simulink model "ANN_model"  (R2023a)
settings: Solver=VariableStepAuto  StartTime=0.0  StopTime=T_e  RelTol=1e-3
libraries: neural x61, spspowerguiLib x1
(part 2 of 2)

== system ANN_model/Custom Neural Network/Layer 4/Delays 1 ==
  "p{4}" : Inport  PortDimensions=10
      mask Display: e = 0.06;c1 = [120 230 180]/255;c2 = ([120 230 180]+0)/(256+128);c3 = ([120 230 180]+128)/(256+128);patch([0 1 1 0],[0 0 1 1],c1);patch([0 1 1 1-e 1-e 0+e],[0 0 1 1-e 0+e 0+e],c2);patch([0 0 1 1-e 0+e 0+e],[0 1 1 1-e 1-e 0+e],c3);plot([0 1 1 0 0],[0 0 1 1 0]);
  mux : Mux  Inputs=1
      mask Display: e = 0.06;c1 = [120 150 230]/255;c2 = ([120 150 230]+0)/383;c3 = ([120 150 230]+128)/383;patch([0 1 1 0],[0 0 1 1],c1);patch([0 1 1 1-e 1-e 0+e],[0 0 1 1-e 0+e 0+e],c2);patch([0 0 1 1-e 0+e 0+e],[0 1 1 1-e 1-e 0+e],c3);plot([0 1 1 0 0],[0 0 1 1 0]);disp('Mux')
  "pd{4,3}" : Outport
      mask Display: e = 0.06;c1 = [120 230 180]/255;c2 = ([120 230 180]+0)/(256+128);c3 = ([120 230 180]+128)/(256+128);patch([0 1 1 0],[0 0 1 1],c1);patch([0 1 1 1-e 1-e 0+e],[0 0 1 1-e 0+e 0+e],c2);patch([0 0 1 1-e 0+e 0+e],[0 1 1 1-e 1-e 0+e],c3);plot([0 1 1 0 0],[0 0 1 1 0]);
  wires:
  "p{4}"/1 -> mux/1
  mux/1 -> "pd{4,3}"/1

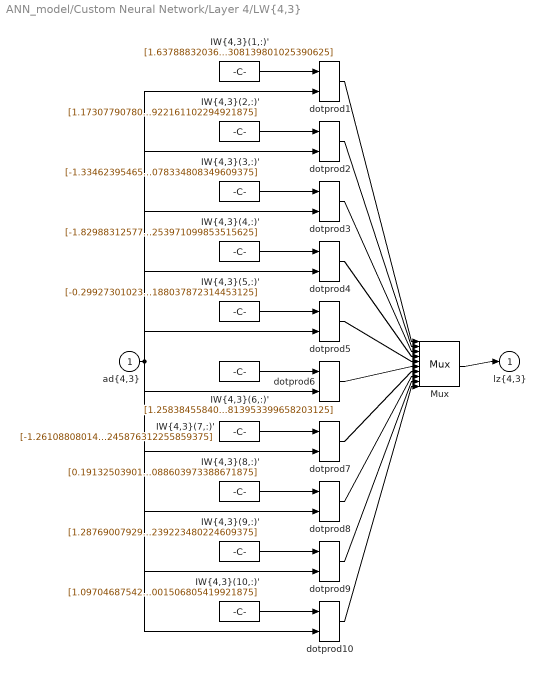
== system ANN_model/Custom Neural Network/Layer 4/LW{4,3} ==
  "ad{4,3}" : Inport  PortDimensions=10
      mask Display: e = 0.06;c1 = [120 230 180]/255;c2 = ([120 230 180]+0)/(256+128);c3 = ([120 230 180]+128)/(256+128);patch([0 1 1 0],[0 0 1 1],c1);patch([0 1 1 1-e 1-e 0+e],[0 0 1 1-e 0+e 0+e],c2);patch([0 0 1 1-e 0+e 0+e],[0 1 1 1-e 1-e 0+e],c3);plot([0 1 1 0 0],[0 0 1 1 0]);
  "IW{4,3}(1,:)'" : Constant  Value=[1.6378883203698550996563199078082107007503509521484375;0.7785713160290177459188498687581159174442291259765625;-3.134049077427762508563091614632867276668548583984375;-4.11400321800767354574190903804264962673187255859375;2.7023166374114051535570979467593133449554443359375;2.178799747279068554917103028856217861175537109375;-1.4904773301039540012169481997261755168437957763671875;-0.434657325226812718543811797644593752920627593994140625;-2.093640295600631251460299608879722654819488525390625;-0.4795777947227544135699872640543617308139801025390625]
      mask Display: e = 0.06;c1 = [120 150 230]/255;c2 = ([120 150 230]+0)/383;c3 = ([120 150 230]+128)/383;patch([0 1 1 0],[0 0 1 1],c1);patch([0 1 1 1-e 1-e 0+e],[0 0 1 1-e 0+e 0+e],c2);patch([0 0 1 1-e 0+e 0+e],[0 1 1 1-e 1-e 0+e],c3);plot([0 1 1 0 0],[0 0 1 1 0]);disp('weights');
  "IW{4,3}(10,:)'" : Constant  Value=[1.0970468754208211326073296731919981539249420166015625;2.598662475604209820545520415180362761020660400390625;3.47585894555124585991734420531429350376129150390625;0.23212021853686748418255092474282719194889068603515625;1.839725276361742434261259404593147337436676025390625;-0.05368765037105353854496314625066588632762432098388671875;2.278073107192821300515106486272998154163360595703125;-0.0687948159269435033369433085681521333754062652587890625;2.86853608695433859310242041829042136669158935546875;-0.328379018423550383953823939009453170001506805419921875]
      mask Display: e = 0.06;c1 = [120 150 230]/255;c2 = ([120 150 230]+0)/383;c3 = ([120 150 230]+128)/383;patch([0 1 1 0],[0 0 1 1],c1);patch([0 1 1 1-e 1-e 0+e],[0 0 1 1-e 0+e 0+e],c2);patch([0 0 1 1-e 0+e 0+e],[0 1 1 1-e 1-e 0+e],c3);plot([0 1 1 0 0],[0 0 1 1 0]);disp('weights');
  "IW{4,3}(2,:)'" : Constant  Value=[1.1730779078006194904304493320523761212825775146484375;-0.93733423397561865808569336877553723752498626708984375;1.4591051184685588371081621517078019678592681884765625;2.1481638705161412161714906687848269939422607421875;-0.97618086283236815692276877598487772047519683837890625;-1.2190160274977539511809254690888337790966033935546875;-1.2100782358443884501042475676513276994228363037109375;-2.800884352505108143560619282652623951435089111328125;0.394266235416011967540583782465546391904354095458984375;0.334912766900543779069465699649299494922161102294921875]
      mask Display: e = 0.06;c1 = [120 150 230]/255;c2 = ([120 150 230]+0)/383;c3 = ([120 150 230]+128)/383;patch([0 1 1 0],[0 0 1 1],c1);patch([0 1 1 1-e 1-e 0+e],[0 0 1 1-e 0+e 0+e],c2);patch([0 0 1 1-e 0+e 0+e],[0 1 1 1-e 1-e 0+e],c3);plot([0 1 1 0 0],[0 0 1 1 0]);disp('weights');
  "IW{4,3}(3,:)'" : Constant  Value=[-1.33462395465049876719376698019914329051971435546875;1.8839799879032177454263319305027835071086883544921875;3.681472741353296829203145534847863018512725830078125;1.707180142477845219417531552608124911785125732421875;-1.44817415107770131044162553735077381134033203125;-3.233967749450946893574609930510632693767547607421875;-1.7261889438801041318782836242462508380413055419921875;-1.873091929612898720591829260229133069515228271484375;0.85833257953746822099816426998586393892765045166015625;1.9157726496007574379376592332846485078334808349609375]
      mask Display: e = 0.06;c1 = [120 150 230]/255;c2 = ([120 150 230]+0)/383;c3 = ([120 150 230]+128)/383;patch([0 1 1 0],[0 0 1 1],c1);patch([0 1 1 1-e 1-e 0+e],[0 0 1 1-e 0+e 0+e],c2);patch([0 0 1 1-e 0+e 0+e],[0 1 1 1-e 1-e 0+e],c3);plot([0 1 1 0 0],[0 0 1 1 0]);disp('weights');
  "IW{4,3}(4,:)'" : Constant  Value=[-1.8298831257738987776662042961106635630130767822265625;-3.1645191260748770645250260713510215282440185546875;-1.2881244508082720923169972593314014375209808349609375;-0.493910555575517218329650859232060611248016357421875;-0.82949048138147596365143954244558699429035186767578125;0.69421918940789650864786608508438803255558013916015625;-1.844328494029690457267633973970077931880950927734375;1.5905908738831155968540542744449339807033538818359375;-1.66302593735684478559733179281465709209442138671875;1.22518832395793797473970698774792253971099853515625]
      mask Display: e = 0.06;c1 = [120 150 230]/255;c2 = ([120 150 230]+0)/383;c3 = ([120 150 230]+128)/383;patch([0 1 1 0],[0 0 1 1],c1);patch([0 1 1 1-e 1-e 0+e],[0 0 1 1-e 0+e 0+e],c2);patch([0 0 1 1-e 0+e 0+e],[0 1 1 1-e 1-e 0+e],c3);plot([0 1 1 0 0],[0 0 1 1 0]);disp('weights');
  "IW{4,3}(5,:)'" : Constant  Value=[-0.299273010230704128442624778472236357629299163818359375;0.50978913541735881853611545011517591774463653564453125;1.097906791329425590930668477085418999195098876953125;2.74186807520239117508253912092186510562896728515625;-0.71921684098344318414319786825217306613922119140625;-2.130424327935024120250773194129578769207000732421875;-0.48862893519710814960177458488033153116703033447265625;1.1831422162157119171155272852047346532344818115234375;0.119131740649917772234545054743648506700992584228515625;0.876286678272823582602768510696478188037872314453125]
      mask Display: e = 0.06;c1 = [120 150 230]/255;c2 = ([120 150 230]+0)/383;c3 = ([120 150 230]+128)/383;patch([0 1 1 0],[0 0 1 1],c1);patch([0 1 1 1-e 1-e 0+e],[0 0 1 1-e 0+e 0+e],c2);patch([0 0 1 1-e 0+e 0+e],[0 1 1 1-e 1-e 0+e],c3);plot([0 1 1 0 0],[0 0 1 1 0]);disp('weights');
  "IW{4,3}(6,:)'" : Constant  Value=[1.258384558409598952266605920158326625823974609375;-2.15265133408728370767448723199777305126190185546875;0.349871100632710818612025605034432373940944671630859375;0.17845212127078780017797043910832144320011138916015625;4.278098869715069696439968538470566272735595703125;-1.2651860443286204738200240171863697469234466552734375;-0.0431755036074752684971400640279171057045459747314453125;0.069751845298305970022312294531730003654956817626953125;-0.320437074873093863391915192551095969974994659423828125;-1.0338974588446216973380842318874783813953399658203125]
      mask Display: e = 0.06;c1 = [120 150 230]/255;c2 = ([120 150 230]+0)/383;c3 = ([120 150 230]+128)/383;patch([0 1 1 0],[0 0 1 1],c1);patch([0 1 1 1-e 1-e 0+e],[0 0 1 1-e 0+e 0+e],c2);patch([0 0 1 1-e 0+e 0+e],[0 1 1 1-e 1-e 0+e],c3);plot([0 1 1 0 0],[0 0 1 1 0]);disp('weights');
  "IW{4,3}(7,:)'" : Constant  Value=[-1.26108808014402828945321743958629667758941650390625;1.2982991534359396013087462051771581172943115234375;-0.35594753368714038277431654933025129139423370361328125;-0.13297185436369274302847998114884831011295318603515625;0.85757738162091190492475334394839592278003692626953125;0.87046854879330248788704693652107380330562591552734375;-3.2413727160328438259284666855819523334503173828125;-0.72558623336712846363383278003311716020107269287109375;0.10456892822654194341591704642269178293645381927490234375;-0.71452112693072178384312564958236180245876312255859375]
      mask Display: e = 0.06;c1 = [120 150 230]/255;c2 = ([120 150 230]+0)/383;c3 = ([120 150 230]+128)/383;patch([0 1 1 0],[0 0 1 1],c1);patch([0 1 1 1-e 1-e 0+e],[0 0 1 1-e 0+e 0+e],c2);patch([0 0 1 1-e 0+e 0+e],[0 1 1 1-e 1-e 0+e],c3);plot([0 1 1 0 0],[0 0 1 1 0]);disp('weights');
  "IW{4,3}(8,:)'" : Constant  Value=[0.1913250390145461443669461232275352813303470611572265625;0.225036006872918414867257297373726032674312591552734375;-6.11190586376111699706825675093568861484527587890625;1.1475267565847711015436516390764154493808746337890625;0.353383174212771600242177783002262003719806671142578125;6.0150369989034704332198089105077087879180908203125;1.605029225551447336073351834784261882305145263671875;0.49390716034623871610875767146353609859943389892578125;1.7498661214561515020449178337003104388713836669921875;2.643356415682688531632038575480692088603973388671875]
      mask Display: e = 0.06;c1 = [120 150 230]/255;c2 = ([120 150 230]+0)/383;c3 = ([120 150 230]+128)/383;patch([0 1 1 0],[0 0 1 1],c1);patch([0 1 1 1-e 1-e 0+e],[0 0 1 1-e 0+e 0+e],c2);patch([0 0 1 1-e 0+e 0+e],[0 1 1 1-e 1-e 0+e],c3);plot([0 1 1 0 0],[0 0 1 1 0]);disp('weights');
  "IW{4,3}(9,:)'" : Constant  Value=[1.287690079297733714014384531765244901180267333984375;-1.444902682493584666900687807356007397174835205078125;-0.29402508747429190183453329154872335493564605712890625;0.0264921265303505355792612618870407459326088428497314453125;-0.12147051106321561653178520145957008935511112213134765625;-0.382550265942154743559200369418249465525150299072265625;-0.7916339264109328865970383048988878726959228515625;-1.8418305905607745831531474323128350079059600830078125;-0.56450801436953546019736904781893827021121978759765625;-0.98129506363542906566266310619539581239223480224609375]
      mask Display: e = 0.06;c1 = [120 150 230]/255;c2 = ([120 150 230]+0)/383;c3 = ([120 150 230]+128)/383;patch([0 1 1 0],[0 0 1 1],c1);patch([0 1 1 1-e 1-e 0+e],[0 0 1 1-e 0+e 0+e],c2);patch([0 0 1 1-e 0+e 0+e],[0 1 1 1-e 1-e 0+e],c3);plot([0 1 1 0 0],[0 0 1 1 0]);disp('weights');
  Mux : Mux  Inputs=10
      mask Display: e = 0.06;c1 = [120 150 230]/255;c2 = ([120 150 230]+0)/383;c3 = ([120 150 230]+128)/383;patch([0 1 1 0],[0 0 1 1],c1);patch([0 1 1 1-e 1-e 0+e],[0 0 1 1-e 0+e 0+e],c2);patch([0 0 1 1-e 0+e 0+e],[0 1 1 1-e 1-e 0+e],c3);plot([0 1 1 0 0],[0 0 1 1 0]);disp('Mux');
  dotprod{1..10} (10 alike) : neural/Weight Functions/dotprod
  "lz{4,3}" : Outport
      mask Display: e = 0.06;c1 = [120 230 180]/255;c2 = ([120 230 180]+0)/(256+128);c3 = ([120 230 180]+128)/(256+128);patch([0 1 1 0],[0 0 1 1],c1);patch([0 1 1 1-e 1-e 0+e],[0 0 1 1-e 0+e 0+e],c2);patch([0 0 1 1-e 0+e 0+e],[0 1 1 1-e 1-e 0+e],c3);plot([0 1 1 0 0],[0 0 1 1 0]);
  wires:
  "IW{4,3}(1,:)'"/1 -> dotprod1/1
  "ad{4,3}"/1 -> dotprod1/2, dotprod2/2, dotprod3/2, dotprod4/2, dotprod5/2, dotprod6/2, dotprod7/2, dotprod8/2, dotprod9/2, dotprod10/2
  dotprod1/1 -> Mux/1
  "IW{4,3}(2,:)'"/1 -> dotprod2/1
  dotprod2/1 -> Mux/2
  "IW{4,3}(3,:)'"/1 -> dotprod3/1
  dotprod3/1 -> Mux/3
  "IW{4,3}(4,:)'"/1 -> dotprod4/1
  dotprod4/1 -> Mux/4
  "IW{4,3}(5,:)'"/1 -> dotprod5/1
  dotprod5/1 -> Mux/5
  "IW{4,3}(6,:)'"/1 -> dotprod6/1
  dotprod6/1 -> Mux/6
  "IW{4,3}(7,:)'"/1 -> dotprod7/1
  dotprod7/1 -> Mux/7
  "IW{4,3}(8,:)'"/1 -> dotprod8/1
  dotprod8/1 -> Mux/8
  "IW{4,3}(9,:)'"/1 -> dotprod9/1
  dotprod9/1 -> Mux/9
  "IW{4,3}(10,:)'"/1 -> dotprod10/1
  dotprod10/1 -> Mux/10
  Mux/1 -> "lz{4,3}"/1

== system ANN_model/Custom Neural Network/Layer 5/Delays 1 ==
  "p{5}" : Inport  PortDimensions=10
      mask Display: e = 0.06;c1 = [120 230 180]/255;c2 = ([120 230 180]+0)/(256+128);c3 = ([120 230 180]+128)/(256+128);patch([0 1 1 0],[0 0 1 1],c1);patch([0 1 1 1-e 1-e 0+e],[0 0 1 1-e 0+e 0+e],c2);patch([0 0 1 1-e 0+e 0+e],[0 1 1 1-e 1-e 0+e],c3);plot([0 1 1 0 0],[0 0 1 1 0]);
  mux : Mux  Inputs=1
      mask Display: e = 0.06;c1 = [120 150 230]/255;c2 = ([120 150 230]+0)/383;c3 = ([120 150 230]+128)/383;patch([0 1 1 0],[0 0 1 1],c1);patch([0 1 1 1-e 1-e 0+e],[0 0 1 1-e 0+e 0+e],c2);patch([0 0 1 1-e 0+e 0+e],[0 1 1 1-e 1-e 0+e],c3);plot([0 1 1 0 0],[0 0 1 1 0]);disp('Mux')
  "pd{5,4}" : Outport
      mask Display: e = 0.06;c1 = [120 230 180]/255;c2 = ([120 230 180]+0)/(256+128);c3 = ([120 230 180]+128)/(256+128);patch([0 1 1 0],[0 0 1 1],c1);patch([0 1 1 1-e 1-e 0+e],[0 0 1 1-e 0+e 0+e],c2);patch([0 0 1 1-e 0+e 0+e],[0 1 1 1-e 1-e 0+e],c3);plot([0 1 1 0 0],[0 0 1 1 0]);
  wires:
  "p{5}"/1 -> mux/1
  mux/1 -> "pd{5,4}"/1

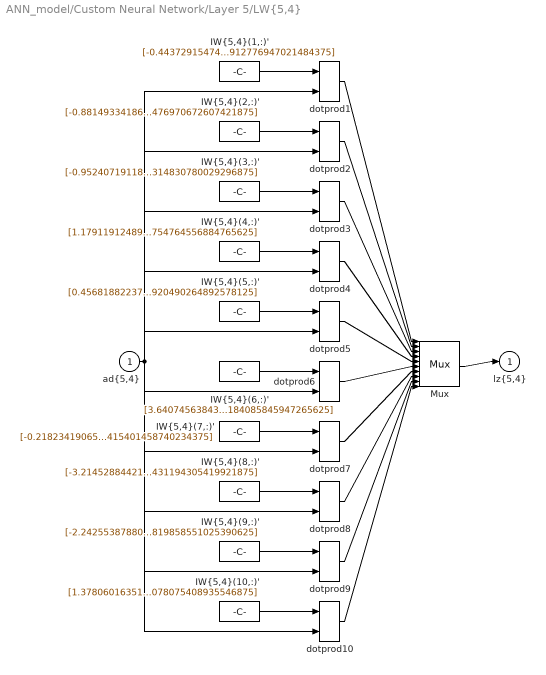
== system ANN_model/Custom Neural Network/Layer 5/LW{5,4} ==
  "ad{5,4}" : Inport  PortDimensions=10
      mask Display: e = 0.06;c1 = [120 230 180]/255;c2 = ([120 230 180]+0)/(256+128);c3 = ([120 230 180]+128)/(256+128);patch([0 1 1 0],[0 0 1 1],c1);patch([0 1 1 1-e 1-e 0+e],[0 0 1 1-e 0+e 0+e],c2);patch([0 0 1 1-e 0+e 0+e],[0 1 1 1-e 1-e 0+e],c3);plot([0 1 1 0 0],[0 0 1 1 0]);
  "IW{5,4}(1,:)'" : Constant  Value=[-0.44372915474945251457228323488379828631877899169921875;-0.08048856572732365766142947904882021248340606689453125;0.3052289457363439595383169944398105144500732421875;-1.592886200917619898831389946280978620052337646484375;-1.0574976706712602148030555326840840280055999755859375;3.0318441877980557563887487049214541912078857421875;2.6572457807686422626147759729065001010894775390625;0.285644863788504010937430166450212709605693817138671875;2.545513406488022045692787287407554686069488525390625;2.398794400241926805250614052056334912776947021484375]
      mask Display: e = 0.06;c1 = [120 150 230]/255;c2 = ([120 150 230]+0)/383;c3 = ([120 150 230]+128)/383;patch([0 1 1 0],[0 0 1 1],c1);patch([0 1 1 1-e 1-e 0+e],[0 0 1 1-e 0+e 0+e],c2);patch([0 0 1 1-e 0+e 0+e],[0 1 1 1-e 1-e 0+e],c3);plot([0 1 1 0 0],[0 0 1 1 0]);disp('weights');
  "IW{5,4}(10,:)'" : Constant  Value=[1.378060163511015456805353096569888293743133544921875;-3.192256397588707717005718222935684025287628173828125;0.7384007420041598379611968994140625;-0.53648879404282912020107687567360699176788330078125;1.9022303694091338144289693445898592472076416015625;-0.409782401405845042585696091919089667499065399169921875;-3.154158555223784521359675636631436645984649658203125;-0.8081742825994415735380016485578380525112152099609375;-1.55348612712726374951444086036644876003265380859375;-2.46842866002258443103301033261232078075408935546875]
      mask Display: e = 0.06;c1 = [120 150 230]/255;c2 = ([120 150 230]+0)/383;c3 = ([120 150 230]+128)/383;patch([0 1 1 0],[0 0 1 1],c1);patch([0 1 1 1-e 1-e 0+e],[0 0 1 1-e 0+e 0+e],c2);patch([0 0 1 1-e 0+e 0+e],[0 1 1 1-e 1-e 0+e],c3);plot([0 1 1 0 0],[0 0 1 1 0]);disp('weights');
  "IW{5,4}(2,:)'" : Constant  Value=[-0.88149334186260841494942042118054814636707305908203125;-0.85890941940042087043849505789694376289844512939453125;-0.401436754943303275577903832527226768434047698974609375;-1.134388757481453513520364140276797115802764892578125;1.6701735466533638163610930860158987343311309814453125;5.81019966239588736556243020459078252315521240234375;3.2797891234911400459850483457557857036590576171875;-0.84227492066083053945391156958066858351230621337890625;-4.382743717276245121183819719590246677398681640625;-1.533996205454193795247874732012860476970672607421875]
      mask Display: e = 0.06;c1 = [120 150 230]/255;c2 = ([120 150 230]+0)/383;c3 = ([120 150 230]+128)/383;patch([0 1 1 0],[0 0 1 1],c1);patch([0 1 1 1-e 1-e 0+e],[0 0 1 1-e 0+e 0+e],c2);patch([0 0 1 1-e 0+e 0+e],[0 1 1 1-e 1-e 0+e],c3);plot([0 1 1 0 0],[0 0 1 1 0]);disp('weights');
  "IW{5,4}(3,:)'" : Constant  Value=[-0.9524071911833764669808033431763760745525360107421875;-1.440247864426563939588277207803912460803985595703125;-0.09067337052139878839085440631606616079807281494140625;3.211647447886596840049833190278150141239166259765625;-3.113299611645719000563303779927082359790802001953125;0.277171941789911946418811794501380063593387603759765625;-0.914863066338964525670007787994109094142913818359375;-0.374506231519017962483530936879105865955352783203125;-2.186056986813969427174697557347826659679412841796875;1.6900012467605936006265210380661301314830780029296875]
      mask Display: e = 0.06;c1 = [120 150 230]/255;c2 = ([120 150 230]+0)/383;c3 = ([120 150 230]+128)/383;patch([0 1 1 0],[0 0 1 1],c1);patch([0 1 1 1-e 1-e 0+e],[0 0 1 1-e 0+e 0+e],c2);patch([0 0 1 1-e 0+e 0+e],[0 1 1 1-e 1-e 0+e],c3);plot([0 1 1 0 0],[0 0 1 1 0]);disp('weights');
  "IW{5,4}(4,:)'" : Constant  Value=[1.1791191248966408355869361912482418119907379150390625;2.031207704811440084569085229304619133472442626953125;0.1341964448633394535459473217997583560645580291748046875;-0.99291564480543481607810463174246251583099365234375;1.2426211118028354096765042413608171045780181884765625;-0.048657784134124505703855589899831102229654788970947265625;-1.18748455604717850775386978057213127613067626953125;-0.659011772753751667863753027631901204586029052734375;-2.255847322448911729253495650482363998889923095703125;-1.068045974981336687648081351653672754764556884765625]
      mask Display: e = 0.06;c1 = [120 150 230]/255;c2 = ([120 150 230]+0)/383;c3 = ([120 150 230]+128)/383;patch([0 1 1 0],[0 0 1 1],c1);patch([0 1 1 1-e 1-e 0+e],[0 0 1 1-e 0+e 0+e],c2);patch([0 0 1 1-e 0+e 0+e],[0 1 1 1-e 1-e 0+e],c3);plot([0 1 1 0 0],[0 0 1 1 0]);disp('weights');
  "IW{5,4}(5,:)'" : Constant  Value=[0.45681882237817117431433189267409034073352813720703125;0.2191730373466506953672450208614463917911052703857421875;-0.1898345875871349786034869566719862632453441619873046875;-1.0656921974338160463702251945505850017070770263671875;1.027043662399730106216111380490474402904510498046875;-2.1421702478158888283132910146377980709075927734375;-1.3597015711374342838979600855964235961437225341796875;-0.32682144504051524602772360594826750457286834716796875;1.7764736465346384619579112040810286998748779296875;-1.7639521181190709331332300280337221920490264892578125]
      mask Display: e = 0.06;c1 = [120 150 230]/255;c2 = ([120 150 230]+0)/383;c3 = ([120 150 230]+128)/383;patch([0 1 1 0],[0 0 1 1],c1);patch([0 1 1 1-e 1-e 0+e],[0 0 1 1-e 0+e 0+e],c2);patch([0 0 1 1-e 0+e 0+e],[0 1 1 1-e 1-e 0+e],c3);plot([0 1 1 0 0],[0 0 1 1 0]);disp('weights');
  "IW{5,4}(6,:)'" : Constant  Value=[3.640745638430612274305531173013150691986083984375;-1.4278802970870696498195684398524463176727294921875;2.9485922999351661388800494023598730564117431640625;-4.41275925093963561351984026259742677211761474609375;4.30707915728340839933707684394903481006622314453125;7.9507897478846825123355301911942660808563232421875;5.16378772799802998605400716769509017467498779296875;-1.0149200969258249660498449884471483528614044189453125;-1.0426889523547802074432411245652474462985992431640625;-0.7695055887698549756947841160581447184085845947265625]
      mask Display: e = 0.06;c1 = [120 150 230]/255;c2 = ([120 150 230]+0)/383;c3 = ([120 150 230]+128)/383;patch([0 1 1 0],[0 0 1 1],c1);patch([0 1 1 1-e 1-e 0+e],[0 0 1 1-e 0+e 0+e],c2);patch([0 0 1 1-e 0+e 0+e],[0 1 1 1-e 1-e 0+e],c3);plot([0 1 1 0 0],[0 0 1 1 0]);disp('weights');
  "IW{5,4}(7,:)'" : Constant  Value=[-0.2182341906556131139183207778842188417911529541015625;0.08219980701825425895012955379570485092699527740478515625;-0.5711068151788041280525476395268924534320831298828125;-0.66723523270064044599081398700946010649204254150390625;0.545520924027612874596115943859331309795379638671875;-0.7218856964225783823252413640148006379604339599609375;-0.354626208286069000141793594593764282763004302978515625;-0.147860903080202887860394866947899572551250457763671875;-1.053609900673512900226569399819709360599517822265625;-0.42586212762334818560105986762209795415401458740234375]
      mask Display: e = 0.06;c1 = [120 150 230]/255;c2 = ([120 150 230]+0)/383;c3 = ([120 150 230]+128)/383;patch([0 1 1 0],[0 0 1 1],c1);patch([0 1 1 1-e 1-e 0+e],[0 0 1 1-e 0+e 0+e],c2);patch([0 0 1 1-e 0+e 0+e],[0 1 1 1-e 1-e 0+e],c3);plot([0 1 1 0 0],[0 0 1 1 0]);disp('weights');
  "IW{5,4}(8,:)'" : Constant  Value=[-3.214528844219887826483272874611429870128631591796875;-2.95747394430882426519247019314207136631011962890625;-2.636002696425631341980988509021699428558349609375;2.571593011677298701300742322928272187709808349609375;2.46358558223354151550665847025811672210693359375;-1.4523946986657636504247648190357722342014312744140625;4.22796835534398951494949869811534881591796875;-1.024206817104519107175519820884801447391510009765625;7.0624384896016412227481851004995405673980712890625;-6.86198307148493835683211727882735431194305419921875]
      mask Display: e = 0.06;c1 = [120 150 230]/255;c2 = ([120 150 230]+0)/383;c3 = ([120 150 230]+128)/383;patch([0 1 1 0],[0 0 1 1],c1);patch([0 1 1 1-e 1-e 0+e],[0 0 1 1-e 0+e 0+e],c2);patch([0 0 1 1-e 0+e 0+e],[0 1 1 1-e 1-e 0+e],c3);plot([0 1 1 0 0],[0 0 1 1 0]);disp('weights');
  "IW{5,4}(9,:)'" : Constant  Value=[-2.24255387880731671401690618949942290782928466796875;0.2131474041792032758646513457279070280492305755615234375;-0.11451107992129962165339662760743522085249423980712890625;-0.058408580933412897195911028802584041841328144073486328125;-6.67116050890009137930292126839049160480499267578125;1.186492100019120865539434817037545144557952880859375;0.66577299553018309818952502610045485198497772216796875;0.0212200176263356195260900705079620820470154285430908203125;1.1533073803396529655174163053743541240692138671875;-0.3195905918601855688621071749366819858551025390625]
      mask Display: e = 0.06;c1 = [120 150 230]/255;c2 = ([120 150 230]+0)/383;c3 = ([120 150 230]+128)/383;patch([0 1 1 0],[0 0 1 1],c1);patch([0 1 1 1-e 1-e 0+e],[0 0 1 1-e 0+e 0+e],c2);patch([0 0 1 1-e 0+e 0+e],[0 1 1 1-e 1-e 0+e],c3);plot([0 1 1 0 0],[0 0 1 1 0]);disp('weights');
  Mux : Mux  Inputs=10
      mask Display: e = 0.06;c1 = [120 150 230]/255;c2 = ([120 150 230]+0)/383;c3 = ([120 150 230]+128)/383;patch([0 1 1 0],[0 0 1 1],c1);patch([0 1 1 1-e 1-e 0+e],[0 0 1 1-e 0+e 0+e],c2);patch([0 0 1 1-e 0+e 0+e],[0 1 1 1-e 1-e 0+e],c3);plot([0 1 1 0 0],[0 0 1 1 0]);disp('Mux');
  dotprod{1..10} (10 alike) : neural/Weight Functions/dotprod
  "lz{5,4}" : Outport
      mask Display: e = 0.06;c1 = [120 230 180]/255;c2 = ([120 230 180]+0)/(256+128);c3 = ([120 230 180]+128)/(256+128);patch([0 1 1 0],[0 0 1 1],c1);patch([0 1 1 1-e 1-e 0+e],[0 0 1 1-e 0+e 0+e],c2);patch([0 0 1 1-e 0+e 0+e],[0 1 1 1-e 1-e 0+e],c3);plot([0 1 1 0 0],[0 0 1 1 0]);
  wires:
  "IW{5,4}(1,:)'"/1 -> dotprod1/1
  "ad{5,4}"/1 -> dotprod1/2, dotprod2/2, dotprod3/2, dotprod4/2, dotprod5/2, dotprod6/2, dotprod7/2, dotprod8/2, dotprod9/2, dotprod10/2
  dotprod1/1 -> Mux/1
  "IW{5,4}(2,:)'"/1 -> dotprod2/1
  dotprod2/1 -> Mux/2
  "IW{5,4}(3,:)'"/1 -> dotprod3/1
  dotprod3/1 -> Mux/3
  "IW{5,4}(4,:)'"/1 -> dotprod4/1
  dotprod4/1 -> Mux/4
  "IW{5,4}(5,:)'"/1 -> dotprod5/1
  dotprod5/1 -> Mux/5
  "IW{5,4}(6,:)'"/1 -> dotprod6/1
  dotprod6/1 -> Mux/6
  "IW{5,4}(7,:)'"/1 -> dotprod7/1
  dotprod7/1 -> Mux/7
  "IW{5,4}(8,:)'"/1 -> dotprod8/1
  dotprod8/1 -> Mux/8
  "IW{5,4}(9,:)'"/1 -> dotprod9/1
  dotprod9/1 -> Mux/9
  "IW{5,4}(10,:)'"/1 -> dotprod10/1
  dotprod10/1 -> Mux/10
  Mux/1 -> "lz{5,4}"/1

== system ANN_model/Custom Neural Network/Layer 6/Delays 1 ==
  "p{6}" : Inport  PortDimensions=10
      mask Display: e = 0.06;c1 = [120 230 180]/255;c2 = ([120 230 180]+0)/(256+128);c3 = ([120 230 180]+128)/(256+128);patch([0 1 1 0],[0 0 1 1],c1);patch([0 1 1 1-e 1-e 0+e],[0 0 1 1-e 0+e 0+e],c2);patch([0 0 1 1-e 0+e 0+e],[0 1 1 1-e 1-e 0+e],c3);plot([0 1 1 0 0],[0 0 1 1 0]);
  mux : Mux  Inputs=1
      mask Display: e = 0.06;c1 = [120 150 230]/255;c2 = ([120 150 230]+0)/383;c3 = ([120 150 230]+128)/383;patch([0 1 1 0],[0 0 1 1],c1);patch([0 1 1 1-e 1-e 0+e],[0 0 1 1-e 0+e 0+e],c2);patch([0 0 1 1-e 0+e 0+e],[0 1 1 1-e 1-e 0+e],c3);plot([0 1 1 0 0],[0 0 1 1 0]);disp('Mux')
  "pd{6,5}" : Outport
      mask Display: e = 0.06;c1 = [120 230 180]/255;c2 = ([120 230 180]+0)/(256+128);c3 = ([120 230 180]+128)/(256+128);patch([0 1 1 0],[0 0 1 1],c1);patch([0 1 1 1-e 1-e 0+e],[0 0 1 1-e 0+e 0+e],c2);patch([0 0 1 1-e 0+e 0+e],[0 1 1 1-e 1-e 0+e],c3);plot([0 1 1 0 0],[0 0 1 1 0]);
  wires:
  "p{6}"/1 -> mux/1
  mux/1 -> "pd{6,5}"/1

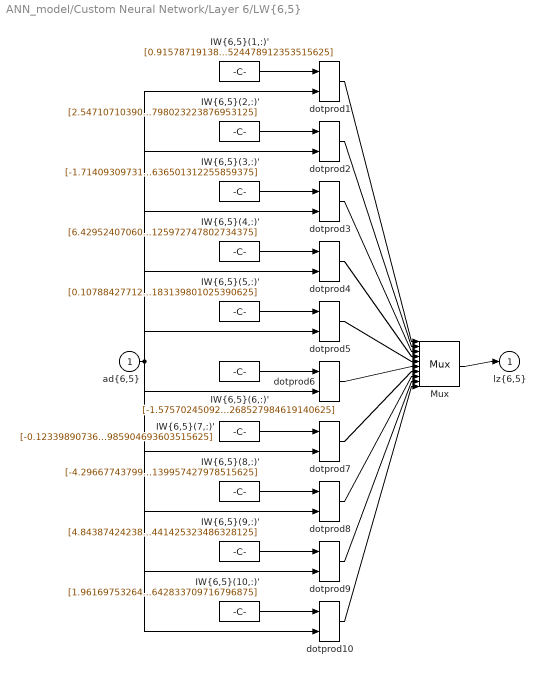
== system ANN_model/Custom Neural Network/Layer 6/LW{6,5} ==
  "ad{6,5}" : Inport  PortDimensions=10
      mask Display: e = 0.06;c1 = [120 230 180]/255;c2 = ([120 230 180]+0)/(256+128);c3 = ([120 230 180]+128)/(256+128);patch([0 1 1 0],[0 0 1 1],c1);patch([0 1 1 1-e 1-e 0+e],[0 0 1 1-e 0+e 0+e],c2);patch([0 0 1 1-e 0+e 0+e],[0 1 1 1-e 1-e 0+e],c3);plot([0 1 1 0 0],[0 0 1 1 0]);
  "IW{6,5}(1,:)'" : Constant  Value=[0.91578719138092001816886522647109813988208770751953125;-1.55629738752322754891110889730043709278106689453125;0.54686041367531867951612412070971913635730743408203125;2.748536495852894834257540424005128443241119384765625;-0.69203669557024827252433851754176430404186248779296875;0.1562862665844011733629059790473547764122486114501953125;-1.1030783465285132205480067568714730441570281982421875;-0.0231553801418886047447376341779090580530464649200439453125;2.756258727328901425579488204675726592540740966796875;-0.48193857734411393867191009121597744524478912353515625]
      mask Display: e = 0.06;c1 = [120 150 230]/255;c2 = ([120 150 230]+0)/383;c3 = ([120 150 230]+128)/383;patch([0 1 1 0],[0 0 1 1],c1);patch([0 1 1 1-e 1-e 0+e],[0 0 1 1-e 0+e 0+e],c2);patch([0 0 1 1-e 0+e 0+e],[0 1 1 1-e 1-e 0+e],c3);plot([0 1 1 0 0],[0 0 1 1 0]);disp('weights');
  "IW{6,5}(10,:)'" : Constant  Value=[1.9616975326464112239222004063776694238185882568359375;-1.0899447413761318426139723669621162116527557373046875;1.2031767189375008886287332643405534327030181884765625;2.03906650011060630589554421021603047847747802734375;2.50600129434051144272643796284683048725128173828125;0.4252173926274915860545888790511526167392730712890625;-2.230662929131254745840351461083628237247467041015625;-0.07630327116655109820353430905015557073056697845458984375;-1.3079000135828906525858883469481952488422393798828125;-1.4236777433878973209147034140187315642833709716796875]
      mask Display: e = 0.06;c1 = [120 150 230]/255;c2 = ([120 150 230]+0)/383;c3 = ([120 150 230]+128)/383;patch([0 1 1 0],[0 0 1 1],c1);patch([0 1 1 1-e 1-e 0+e],[0 0 1 1-e 0+e 0+e],c2);patch([0 0 1 1-e 0+e 0+e],[0 1 1 1-e 1-e 0+e],c3);plot([0 1 1 0 0],[0 0 1 1 0]);disp('weights');
  "IW{6,5}(2,:)'" : Constant  Value=[2.547107103900183577849247740232385694980621337890625;-1.2370150361727978438608488431782461702823638916015625;0.989661630898456490257331097382120788097381591796875;-2.862189591738488303462872863747179508209228515625;-1.8002999427067949422820447580306790769100189208984375;-1.071065879591814873350585912703536450862884521484375;-0.357942338977107532560495428697322495281696319580078125;-0.474367748873758376948472914591548033058643341064453125;-2.868888218359867181561639881692826747894287109375;0.59131397526320317314940666619804687798023223876953125]
      mask Display: e = 0.06;c1 = [120 150 230]/255;c2 = ([120 150 230]+0)/383;c3 = ([120 150 230]+128)/383;patch([0 1 1 0],[0 0 1 1],c1);patch([0 1 1 1-e 1-e 0+e],[0 0 1 1-e 0+e 0+e],c2);patch([0 0 1 1-e 0+e 0+e],[0 1 1 1-e 1-e 0+e],c3);plot([0 1 1 0 0],[0 0 1 1 0]);disp('weights');
  "IW{6,5}(3,:)'" : Constant  Value=[-1.7140930973196975006800357732572592794895172119140625;0.1535266433030496868727965420475811697542667388916015625;-1.584619785562153548852393214474432170391082763671875;0.72668287956691279827481366737629286944866180419921875;0.032179627298217404474112157686249702237546443939208984375;-0.225522758623212860040752048007561825215816497802734375;0.1636206551172376955083365146492724306881427764892578125;-0.00968246359250476452962264062307440326549112796783447265625;0.34861364819909079759696624023490585386753082275390625;0.56444552208853548957989687551162205636501312255859375]
      mask Display: e = 0.06;c1 = [120 150 230]/255;c2 = ([120 150 230]+0)/383;c3 = ([120 150 230]+128)/383;patch([0 1 1 0],[0 0 1 1],c1);patch([0 1 1 1-e 1-e 0+e],[0 0 1 1-e 0+e 0+e],c2);patch([0 0 1 1-e 0+e 0+e],[0 1 1 1-e 1-e 0+e],c3);plot([0 1 1 0 0],[0 0 1 1 0]);disp('weights');
  "IW{6,5}(4,:)'" : Constant  Value=[6.429524070607516961217697826214134693145751953125;-2.74197592228397990510302406619302928447723388671875;0.256586162676969486984290824693744070827960968017578125;0.97924535689561176265982567201717756688594818115234375;-0.048702914274068032085551749332807958126068115234375;1.1089893356618187869599978512269444763660430908203125;0.18199381171876527485409269502270035445690155029296875;-1.6772060408506941353579122733208350837230682373046875;-1.4422098408455801266114804093376733362674713134765625;-0.70564252785975634107984433285309933125972747802734375]
      mask Display: e = 0.06;c1 = [120 150 230]/255;c2 = ([120 150 230]+0)/383;c3 = ([120 150 230]+128)/383;patch([0 1 1 0],[0 0 1 1],c1);patch([0 1 1 1-e 1-e 0+e],[0 0 1 1-e 0+e 0+e],c2);patch([0 0 1 1-e 0+e 0+e],[0 1 1 1-e 1-e 0+e],c3);plot([0 1 1 0 0],[0 0 1 1 0]);disp('weights');
  "IW{6,5}(5,:)'" : Constant  Value=[0.1078842771219472862487265274467063136398792266845703125;-3.047905569663435176863686137949116528034210205078125;1.4335200662792810799572862379136495292186737060546875;2.320543171533404613882112244027666747570037841796875;-2.5113045243300557984866827609948813915252685546875;-0.903995819636644881711617927066981792449951171875;-0.219366015134729475111186047797673381865024566650390625;-0.10142263428830318450213354708466795273125171661376953125;2.221543434905808300783291997504420578479766845703125;0.82013893697738604604552392629557289183139801025390625]
      mask Display: e = 0.06;c1 = [120 150 230]/255;c2 = ([120 150 230]+0)/383;c3 = ([120 150 230]+128)/383;patch([0 1 1 0],[0 0 1 1],c1);patch([0 1 1 1-e 1-e 0+e],[0 0 1 1-e 0+e 0+e],c2);patch([0 0 1 1-e 0+e 0+e],[0 1 1 1-e 1-e 0+e],c3);plot([0 1 1 0 0],[0 0 1 1 0]);disp('weights');
  "IW{6,5}(6,:)'" : Constant  Value=[-1.5757024509265722400641607237048447132110595703125;-1.4788344867066933741028833537711761891841888427734375;-3.442514062005115338394034552038647234439849853515625;-0.2382520312311966759200032583976280875504016876220703125;1.497684775384521049801378467236645519733428955078125;4.13624333301294111464585512294434010982513427734375;2.19992795031512766712467055185697972774505615234375;4.1038456995736734000956857926212251186370849609375;-2.899853285371538635928345684078522026538848876953125;-0.44303102669186034123782746974029578268527984619140625]
      mask Display: e = 0.06;c1 = [120 150 230]/255;c2 = ([120 150 230]+0)/383;c3 = ([120 150 230]+128)/383;patch([0 1 1 0],[0 0 1 1],c1);patch([0 1 1 1-e 1-e 0+e],[0 0 1 1-e 0+e 0+e],c2);patch([0 0 1 1-e 0+e 0+e],[0 1 1 1-e 1-e 0+e],c3);plot([0 1 1 0 0],[0 0 1 1 0]);disp('weights');
  "IW{6,5}(7,:)'" : Constant  Value=[-0.12339890736810400773126872309148893691599369049072265625;0.3604110063402554686717849108390510082244873046875;0.2236305260972994701784699600466410629451274871826171875;-3.001743632204584510958511600620113313198089599609375;-3.175338986178352751466036352212540805339813232421875;0.07216064110590635072295384588869637809693813323974609375;2.434394811718374906917006228468380868434906005859375;1.433225119095112187750373777817003428936004638671875;1.111417931855736451751681670430116355419158935546875;1.0265050603734791057064512642682529985904693603515625]
      mask Display: e = 0.06;c1 = [120 150 230]/255;c2 = ([120 150 230]+0)/383;c3 = ([120 150 230]+128)/383;patch([0 1 1 0],[0 0 1 1],c1);patch([0 1 1 1-e 1-e 0+e],[0 0 1 1-e 0+e 0+e],c2);patch([0 0 1 1-e 0+e 0+e],[0 1 1 1-e 1-e 0+e],c3);plot([0 1 1 0 0],[0 0 1 1 0]);disp('weights');
  "IW{6,5}(8,:)'" : Constant  Value=[-4.29667743799932200232660761685110628604888916015625;-0.760910851621952932788417456322349607944488525390625;1.7104070974715936959142936757416464388370513916015625;-0.917203166474953146547477444983087480068206787109375;0.210528617658457706252050911643891595304012298583984375;0.2378764197373051392236931178558734245598316192626953125;1.7950791510260295513745631978963501751422882080078125;0.428901383228725341378861912744469009339809417724609375;1.338085305387935353138573191245086491107940673828125;-3.301177106428254237613373334170319139957427978515625]
      mask Display: e = 0.06;c1 = [120 150 230]/255;c2 = ([120 150 230]+0)/383;c3 = ([120 150 230]+128)/383;patch([0 1 1 0],[0 0 1 1],c1);patch([0 1 1 1-e 1-e 0+e],[0 0 1 1-e 0+e 0+e],c2);patch([0 0 1 1-e 0+e 0+e],[0 1 1 1-e 1-e 0+e],c3);plot([0 1 1 0 0],[0 0 1 1 0]);disp('weights');
  "IW{6,5}(9,:)'" : Constant  Value=[4.84387424238289643341204282478429377079010009765625;-2.376262714953159882469435615348629653453826904296875;0.17314897923240046839765682307188399136066436767578125;0.1592364945987707336438887750773574225604534149169921875;-0.66603962705694097490294325325521640479564666748046875;0.87152140202362204934871670047868974506855010986328125;-0.09926220800599694360499825052102096378803253173828125;-1.50811297228336993470065863220952451229095458984375;-0.39957998898942903576170238011400215327739715576171875;0.69693437264745228265638843367923982441425323486328125]
      mask Display: e = 0.06;c1 = [120 150 230]/255;c2 = ([120 150 230]+0)/383;c3 = ([120 150 230]+128)/383;patch([0 1 1 0],[0 0 1 1],c1);patch([0 1 1 1-e 1-e 0+e],[0 0 1 1-e 0+e 0+e],c2);patch([0 0 1 1-e 0+e 0+e],[0 1 1 1-e 1-e 0+e],c3);plot([0 1 1 0 0],[0 0 1 1 0]);disp('weights');
  Mux : Mux  Inputs=10
      mask Display: e = 0.06;c1 = [120 150 230]/255;c2 = ([120 150 230]+0)/383;c3 = ([120 150 230]+128)/383;patch([0 1 1 0],[0 0 1 1],c1);patch([0 1 1 1-e 1-e 0+e],[0 0 1 1-e 0+e 0+e],c2);patch([0 0 1 1-e 0+e 0+e],[0 1 1 1-e 1-e 0+e],c3);plot([0 1 1 0 0],[0 0 1 1 0]);disp('Mux');
  dotprod{1..10} (10 alike) : neural/Weight Functions/dotprod
  "lz{6,5}" : Outport
      mask Display: e = 0.06;c1 = [120 230 180]/255;c2 = ([120 230 180]+0)/(256+128);c3 = ([120 230 180]+128)/(256+128);patch([0 1 1 0],[0 0 1 1],c1);patch([0 1 1 1-e 1-e 0+e],[0 0 1 1-e 0+e 0+e],c2);patch([0 0 1 1-e 0+e 0+e],[0 1 1 1-e 1-e 0+e],c3);plot([0 1 1 0 0],[0 0 1 1 0]);
  wires:
  "IW{6,5}(1,:)'"/1 -> dotprod1/1
  "ad{6,5}"/1 -> dotprod1/2, dotprod2/2, dotprod3/2, dotprod4/2, dotprod5/2, dotprod6/2, dotprod7/2, dotprod8/2, dotprod9/2, dotprod10/2
  dotprod1/1 -> Mux/1
  "IW{6,5}(2,:)'"/1 -> dotprod2/1
  dotprod2/1 -> Mux/2
  "IW{6,5}(3,:)'"/1 -> dotprod3/1
  dotprod3/1 -> Mux/3
  "IW{6,5}(4,:)'"/1 -> dotprod4/1
  dotprod4/1 -> Mux/4
  "IW{6,5}(5,:)'"/1 -> dotprod5/1
  dotprod5/1 -> Mux/5
  "IW{6,5}(6,:)'"/1 -> dotprod6/1
  dotprod6/1 -> Mux/6
  "IW{6,5}(7,:)'"/1 -> dotprod7/1
  dotprod7/1 -> Mux/7
  "IW{6,5}(8,:)'"/1 -> dotprod8/1
  dotprod8/1 -> Mux/8
  "IW{6,5}(9,:)'"/1 -> dotprod9/1
  dotprod9/1 -> Mux/9
  "IW{6,5}(10,:)'"/1 -> dotprod10/1
  dotprod10/1 -> Mux/10
  Mux/1 -> "lz{6,5}"/1

== system ANN_model/Custom Neural Network/Layer 7/Delays 1 ==
  "p{7}" : Inport  PortDimensions=10
      mask Display: e = 0.06;c1 = [120 230 180]/255;c2 = ([120 230 180]+0)/(256+128);c3 = ([120 230 180]+128)/(256+128);patch([0 1 1 0],[0 0 1 1],c1);patch([0 1 1 1-e 1-e 0+e],[0 0 1 1-e 0+e 0+e],c2);patch([0 0 1 1-e 0+e 0+e],[0 1 1 1-e 1-e 0+e],c3);plot([0 1 1 0 0],[0 0 1 1 0]);
  mux : Mux  Inputs=1
      mask Display: e = 0.06;c1 = [120 150 230]/255;c2 = ([120 150 230]+0)/383;c3 = ([120 150 230]+128)/383;patch([0 1 1 0],[0 0 1 1],c1);patch([0 1 1 1-e 1-e 0+e],[0 0 1 1-e 0+e 0+e],c2);patch([0 0 1 1-e 0+e 0+e],[0 1 1 1-e 1-e 0+e],c3);plot([0 1 1 0 0],[0 0 1 1 0]);disp('Mux')
  "pd{7,6}" : Outport
      mask Display: e = 0.06;c1 = [120 230 180]/255;c2 = ([120 230 180]+0)/(256+128);c3 = ([120 230 180]+128)/(256+128);patch([0 1 1 0],[0 0 1 1],c1);patch([0 1 1 1-e 1-e 0+e],[0 0 1 1-e 0+e 0+e],c2);patch([0 0 1 1-e 0+e 0+e],[0 1 1 1-e 1-e 0+e],c3);plot([0 1 1 0 0],[0 0 1 1 0]);
  wires:
  "p{7}"/1 -> mux/1
  mux/1 -> "pd{7,6}"/1

== system ANN_model/Custom Neural Network/Layer 7/LW{7,6} ==
  "ad{7,6}" : Inport  PortDimensions=10
      mask Display: e = 0.06;c1 = [120 230 180]/255;c2 = ([120 230 180]+0)/(256+128);c3 = ([120 230 180]+128)/(256+128);patch([0 1 1 0],[0 0 1 1],c1);patch([0 1 1 1-e 1-e 0+e],[0 0 1 1-e 0+e 0+e],c2);patch([0 0 1 1-e 0+e 0+e],[0 1 1 1-e 1-e 0+e],c3);plot([0 1 1 0 0],[0 0 1 1 0]);
  "IW{7,6}(1,:)'" : Constant  Value=[0.45870269916964556689009668843937106430530548095703125;0.428143151563848578522453180994489230215549468994140625;0.71355469509929225768729565970716066658496856689453125;1.3176188360152185641283040240523405373096466064453125;-0.51340107680674107459850574741722084581851959228515625;-0.1598521866598419938210184909621602855622768402099609375;0.61696595877213178393816406241967342793941497802734375;-0.958291455027545424627533066086471080780029296875;-1.92375706688332126503837571362964808940887451171875;1.5492398687950010849334603335591964423656463623046875]
      mask Display: e = 0.06;c1 = [120 150 230]/255;c2 = ([120 150 230]+0)/383;c3 = ([120 150 230]+128)/383;patch([0 1 1 0],[0 0 1 1],c1);patch([0 1 1 1-e 1-e 0+e],[0 0 1 1-e 0+e 0+e],c2);patch([0 0 1 1-e 0+e 0+e],[0 1 1 1-e 1-e 0+e],c3);plot([0 1 1 0 0],[0 0 1 1 0]);disp('weights');
  Mux : Mux  Inputs=1
      mask Display: e = 0.06;c1 = [120 150 230]/255;c2 = ([120 150 230]+0)/383;c3 = ([120 150 230]+128)/383;patch([0 1 1 0],[0 0 1 1],c1);patch([0 1 1 1-e 1-e 0+e],[0 0 1 1-e 0+e 0+e],c2);patch([0 0 1 1-e 0+e 0+e],[0 1 1 1-e 1-e 0+e],c3);plot([0 1 1 0 0],[0 0 1 1 0]);disp('Mux');
  dotprod1 : neural/Weight Functions/dotprod
  "lz{7,6}" : Outport
      mask Display: e = 0.06;c1 = [120 230 180]/255;c2 = ([120 230 180]+0)/(256+128);c3 = ([120 230 180]+128)/(256+128);patch([0 1 1 0],[0 0 1 1],c1);patch([0 1 1 1-e 1-e 0+e],[0 0 1 1-e 0+e 0+e],c2);patch([0 0 1 1-e 0+e 0+e],[0 1 1 1-e 1-e 0+e],c3);plot([0 1 1 0 0],[0 0 1 1 0]);
  wires:
  "IW{7,6}(1,:)'"/1 -> dotprod1/1
  "ad{7,6}"/1 -> dotprod1/2
  dotprod1/1 -> Mux/1
  Mux/1 -> "lz{7,6}"/1

== matlab function ANN_model/MATLAB Function ==
  data: u input; y output; v input; w input
function y = fcn(u,v,w)


all=[u;v;w];

y = all;
